simulink model "single_synapse_electrical"  (R2024a)
settings: Solver=FixedStepAuto  StartTime=0.0  StopTime=4  FixedStep=0.0001  RelTol=1e-3
libraries: fl_lib x65, nesl_utility x5
settings Model: Creator=Aleksandar Kežić  LastModifiedBy=Aleksandar Kežić

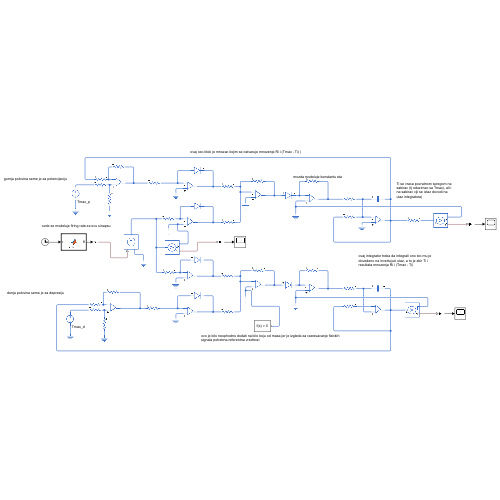
[thumbnail: Simulink's stored preview of the top-level diagram]
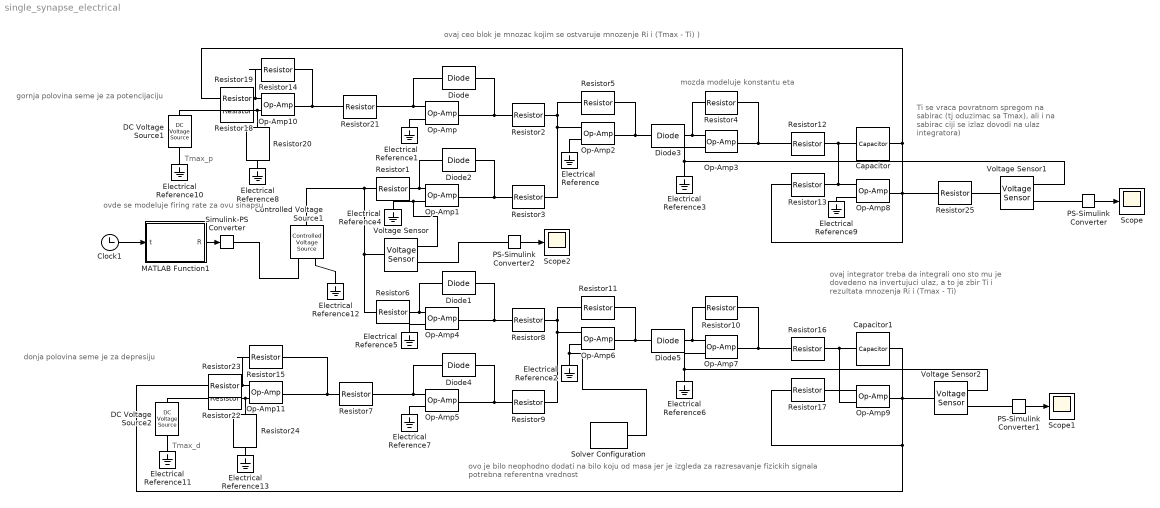
== system single_synapse_electrical ==
  note: mozda modeluje konstantu eta
  note: Ti se vraca povratnom spregom na sabirac (tj oduzimac sa Tmax), ali i na sabirac ciji se izlaz dovodi na ulaz integratora)
  note: ovaj ceo blok je mnozac kojim se ostvaruje mnozenje Ri i (Tmax - Ti) )
  note: ovaj integrator treba da integrali ono sto mu je dovedeno na invertujuci ulaz, a to je zbir Ti i rezultata mnozenja Ri i (Tmax - Ti)
  note: Tmax_p
  note: ovo je bilo neophodno dodati na bilo koju od masa jer je izgleda za razresavanje fizickih signala potrebna referentna vrednost
  note: ovde se modeluje firing rate za ovu sinapsu
  note: gornja polovina seme je za potencijaciju
  note: donja polovina seme je za depresiju
  note: Tmax_d
  Capacitor : fl_lib/Electrical/Electrical Elements/Capacitor  c=1e-7 F  r=1e-6 Ohm  g=0 1/Ohm  i_specify=off  i_priority=None  i=0 A  i_nominal_specify=off  i_nominal_value=1  i_nominal_unit=A  v_specify=off  v_priority=None  v=0 V  v_nominal_specify=off  v_nominal_value=1  v_nominal_unit=V  vc_specify=off  vc_priority=High  vc=0 V  vc_nominal_specify=off  vc_nominal_value=1  vc_nominal_unit=V
  Capacitor1 : fl_lib/Electrical/Electrical Elements/Capacitor  c=1e-7 F  r=1e-6 Ohm  g=0 1/Ohm  i_specify=off  i_priority=None  i=0 A  i_nominal_specify=off  i_nominal_value=1  i_nominal_unit=A  v_specify=off  v_priority=None  v=0 V  v_nominal_specify=off  v_nominal_value=1  v_nominal_unit=V  vc_specify=off  vc_priority=High  vc=0 V  vc_nominal_specify=off  vc_nominal_value=1  vc_nominal_unit=V
  Clock1 : Clock
  Controlled Voltage Source1 : fl_lib/Electrical/Electrical Sources/Controlled Voltage Source
  DC Voltage Source1 : fl_lib/Electrical/Electrical Sources/DC Voltage Source  v0=2.2 V
  DC Voltage Source2 : fl_lib/Electrical/Electrical Sources/DC Voltage Source  v0=2 V
  Diode{,1..5} (6 alike) : fl_lib/Electrical/Electrical Elements/Diode  Vf=0.6 V  Ron=0.3 Ohm  Goff=1e-8 1/Ohm  i_specify=off  i_priority=None  i=0 A  i_nominal_specify=off  i_nominal_value=1  i_nominal_unit=A  v_specify=off  v_priority=None  v=0 V  v_nominal_specify=off  v_nominal_value=1  v_nominal_unit=V
  Electrical Reference{,1..13} (14 alike) : fl_lib/Electrical/Electrical Elements/Electrical Reference
  MATLAB Function1 : MATLAB Function  TreatAsAtomicUnit=on
  Op-Amp{,1..11} (12 alike) : fl_lib/Electrical/Electrical Elements/Op-Amp  outI_specify=off  outI_priority=None  outI=0 A  outI_nominal_specify=off  outI_nominal_value=1  outI_nominal_unit=A
  PS-Simulink Converter : nesl_utility/PS-Simulink Converter  PhysicalDomain=network_engine_domain  SubClassName=ps_output  LeftPortType=input  RightPortType=output  PseudoPeriodic=off  Frequencies=[]  VectorFormat=inherit  Unit=inherit  AffineConversion=off
  PS-Simulink Converter1 : nesl_utility/PS-Simulink Converter  PhysicalDomain=network_engine_domain  SubClassName=ps_output  LeftPortType=input  RightPortType=output  PseudoPeriodic=off  Frequencies=[]  VectorFormat=inherit  Unit=inherit  AffineConversion=off
  PS-Simulink Converter2 : nesl_utility/PS-Simulink Converter  PhysicalDomain=network_engine_domain  SubClassName=ps_output  LeftPortType=input  RightPortType=output  PseudoPeriodic=off  Frequencies=[]  VectorFormat=inherit  Unit=inherit  AffineConversion=off
  Resistor{1..11,14..24} (22 alike) : fl_lib/Electrical/Electrical Elements/Resistor  R=1 Ohm  i_specify=off  i_priority=None  i=0 A  i_nominal_specify=off  i_nominal_value=1  i_nominal_unit=A  v_specify=off  v_priority=None  v=0 V  v_nominal_specify=off  v_nominal_value=1  v_nominal_unit=V
  Resistor12 : fl_lib/Electrical/Electrical Elements/Resistor  R=1 MOhm  i_specify=off  i_priority=None  i=0 A  i_nominal_specify=off  i_nominal_value=1  i_nominal_unit=A  v_specify=off  v_priority=None  v=0 V  v_nominal_specify=off  v_nominal_value=1  v_nominal_unit=V
  Resistor13 : fl_lib/Electrical/Electrical Elements/Resistor  R=1 MOhm  i_specify=off  i_priority=None  i=0 A  i_nominal_specify=off  i_nominal_value=1  i_nominal_unit=A  v_specify=off  v_priority=None  v=0 V  v_nominal_specify=off  v_nominal_value=1  v_nominal_unit=V
  Resistor25 : fl_lib/Electrical/Electrical Elements/Resistor  R=1 kOhm  i_specify=off  i_priority=None  i=0 A  i_nominal_specify=off  i_nominal_value=1  i_nominal_unit=A  v_specify=off  v_priority=None  v=0 V  v_nominal_specify=off  v_nominal_value=1  v_nominal_unit=V
  Scope : Scope
  Scope1 : Scope
  Scope2 : Scope
  Simulink-PS Converter : nesl_utility/Simulink-PS Converter  PhysicalDomain=network_engine_domain  SubClassName=ps_input  LeftPortType=input  RightPortType=output  PseudoPeriodic=off  Frequencies=[]  NoiseDistribution=none  NoiseParameters=[]  Unit=1  AffineConversion=off  FilteringAndDerivatives=provide  SimscapeFilterOrder=1  InputFilterTimeConstant=0.001  UdotUserProvided=0
  Solver Configuration : nesl_utility/Solver Configuration  PhysicalDomain=network_engine_domain  SubClassName=solver  LeftPortType=input  RightPortType=generic  Tones=[]  Harmonics=[]  SimulateNoise=off  Profile=off  UseLocalSampling=off  EnableSwitchedLinearOptims=on  FrequencyDomain=off  UseCCode=off  RelTol=0.001  AbsTol=0.001  MinStep=1e-09  ToWorkspace=off  RevertToSquareIcSolve=off  NumHomotopyIterations=100  PhasorMode=off  PhasorModeNumHarmonics=1  ConsistencySolver=NEWTON_XTOL_AFTER_FTOL  IndexReductionMethod=DerivativeReplacement  DoDC=off  ResidualTolerance=1e-09  ConsistencyTolSource=GLOBAL  ConsistencyAbsTol=0.001  ConsistencyRelTol=0.001  ConsistencyTolFactor=0.001  UseLocalSolver=off  LocalSolverChoice=NE_BACKWARD_EULER_ADVANCER  ResolveIndetEquations=on  FunctionEvalNumThread=1  LocalSolverSampleTime=0.001  DoFixedCost=off  MaxNonlinIter=3  MaxModeIter=2  ComputeImpulses=off  ImpulseIterations=2  LinearAlgebra=auto  LinearAlgebraNumThread=0  EquationFormulation=NE_TIME_EF  DelaysMemoryBudget=1024  AutomaticFiltering=on  FilteringTimeConstant=0.001  PartitionStorageMethod=AS_NEEDED  PartitionMemoryBudget=1024  PartitionMethod=ROBUST  MultibodyUseLocalSolver=off  MultibodyLocalSolverChoice=ODE1  MultibodyLocalSolverSampleTime=0.001
  Voltage Sensor : fl_lib/Electrical/Electrical Sensors/Voltage Sensor
  Voltage Sensor1 : fl_lib/Electrical/Electrical Sensors/Voltage Sensor
  Voltage Sensor2 : fl_lib/Electrical/Electrical Sensors/Voltage Sensor
  wires:
  PS-Simulink Converter/1 -> Scope/1
  PS-Simulink Converter1/1 -> Scope1/1
  PS-Simulink Converter2/1 -> Scope2/1
  Clock1/1 -> MATLAB Function1/1(t)
  MATLAB Function1/1(R) -> Simulink-PS Converter/1
  connections:
  Diode/LConn1 -- Resistor21/RConn1 -- Op-Amp/LConn2
  Op-Amp/LConn1 -- Electrical Reference1/LConn1
  Diode/RConn1 -- Op-Amp/RConn1 -- Resistor2/LConn1
  Resistor1/RConn1 -- Diode2/LConn1 -- Op-Amp1/LConn2
  Op-Amp1/LConn1 -- Electrical Reference4/LConn1 -- Voltage Sensor/RConn2
  Diode2/RConn1 -- Op-Amp1/RConn1 -- Resistor3/LConn1
  Resistor2/RConn1 -- Op-Amp2/LConn2 -- Resistor3/RConn1 -- Resistor5/LConn1
  Op-Amp2/LConn1 -- Electrical Reference/LConn1
  Resistor5/RConn1 -- Op-Amp2/RConn1 -- Diode3/LConn1
  Op-Amp3/LConn2 -- Resistor4/LConn1 -- Diode3/RConn1
  Resistor4/RConn1 -- Op-Amp3/RConn1 -- Resistor12/LConn1
  Op-Amp3/LConn1 -- Electrical Reference3/LConn1 -- Voltage Sensor1/RConn2
  Diode4/RConn1 -- Op-Amp5/RConn1 -- Resistor9/LConn1
  Resistor8/RConn1 -- Resistor11/LConn1 -- Op-Amp6/LConn2 -- Resistor9/RConn1
  Diode1/RConn1 -- Op-Amp4/RConn1 -- Resistor8/LConn1
  Resistor7/RConn1 -- Diode4/LConn1 -- Op-Amp5/LConn2
  Resistor11/RConn1 -- Op-Amp6/RConn1 -- Diode5/LConn1
  Op-Amp7/LConn2 -- Resistor10/LConn1 -- Diode5/RConn1
  Resistor6/RConn1 -- Diode1/LConn1 -- Op-Amp4/LConn2
  Resistor10/RConn1 -- Resistor16/LConn1 -- Op-Amp7/RConn1
  Op-Amp7/LConn1 -- Voltage Sensor2/RConn2 -- Electrical Reference6/LConn1
  Op-Amp4/LConn1 -- Electrical Reference5/LConn1
  Op-Amp6/LConn1 -- Solver Configuration/RConn1 -- Electrical Reference2/LConn1
  Op-Amp5/LConn1 -- Electrical Reference7/LConn1
  Resistor1/LConn1 -- Controlled Voltage Source1/LConn1 -- Voltage Sensor/LConn1 -- Resistor6/LConn1
  Resistor12/RConn1 -- Resistor13/RConn1 -- Op-Amp8/LConn2 -- Capacitor/LConn1
  Capacitor/RConn1 -- Resistor19/LConn1 -- Resistor25/LConn1 -- Resistor13/LConn1 -- Op-Amp8/RConn1
  Electrical Reference10/LConn1 -- DC Voltage Source1/RConn1
  Resistor16/RConn1 -- Op-Amp9/LConn1 -- Capacitor1/LConn1
  Capacitor1/RConn1 -- Resistor23/LConn1 -- Resistor17/LConn1 -- Voltage Sensor2/LConn1 -- Op-Amp9/RConn1
  Voltage Sensor1/RConn1 -- PS-Simulink Converter/LConn1
  Voltage Sensor2/RConn1 -- PS-Simulink Converter1/LConn1
  Voltage Sensor/RConn1 -- PS-Simulink Converter2/LConn1
  Electrical Reference12/LConn1 -- Controlled Voltage Source1/RConn2
  Controlled Voltage Source1/RConn1 -- Simulink-PS Converter/RConn1
  Op-Amp9/LConn2 -- Resistor17/RConn1
  Op-Amp10/LConn1 -- Resistor20/LConn1 -- Resistor18/RConn1
  Resistor19/RConn1 -- Resistor14/LConn1 -- Op-Amp10/LConn2
  Resistor18/LConn1 -- DC Voltage Source1/LConn1
  Resistor20/RConn1 -- Electrical Reference8/LConn1
  Op-Amp10/RConn1 -- Resistor21/LConn1 -- Resistor14/RConn1
  Resistor15/RConn1 -- Op-Amp11/RConn1 -- Resistor7/LConn1
  Op-Amp11/LConn1 -- Resistor24/LConn1 -- Resistor22/RConn1
  Resistor23/RConn1 -- Resistor15/LConn1 -- Op-Amp11/LConn2
  Resistor24/RConn1 -- Electrical Reference13/LConn1
  Electrical Reference11/LConn1 -- DC Voltage Source2/RConn1
  Resistor22/LConn1 -- DC Voltage Source2/LConn1
  Op-Amp8/LConn1 -- Electrical Reference9/LConn1
  Resistor25/RConn1 -- Voltage Sensor1/LConn1

== matlab function single_synapse_electrical/MATLAB Function1 ==
  data: t input; R output
function R = R_func(t)
    alpha = 7.5;
    sigma = 0.9/(3*sqrt(2));
    v = 0.5;
    x0 = 0.4; % place field center of a single synapse
    R = alpha * exp(-((v*t - x0)/sigma)^2);
end
